simulink subsystem "Three_PhasePRController"  (R2023b)
settings: Solver=VariableStepAuto  StartTime=0.0  StopTime=10.0  RelTol=1e-3
undefined symbols (not defined in the file): prCurrentCtrl
settings Model: Creator=Veimar  LastModifiedBy=Veimar

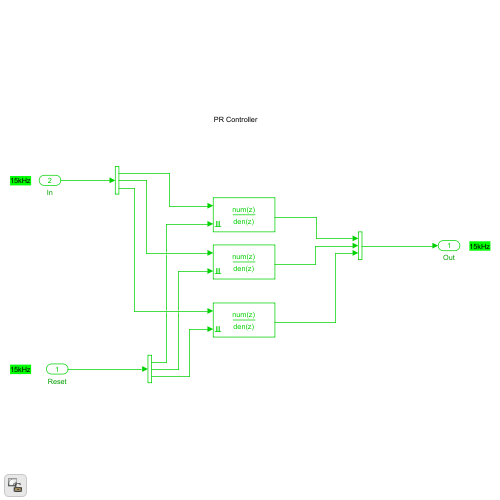
[thumbnail: Simulink's stored preview of the top-level diagram]
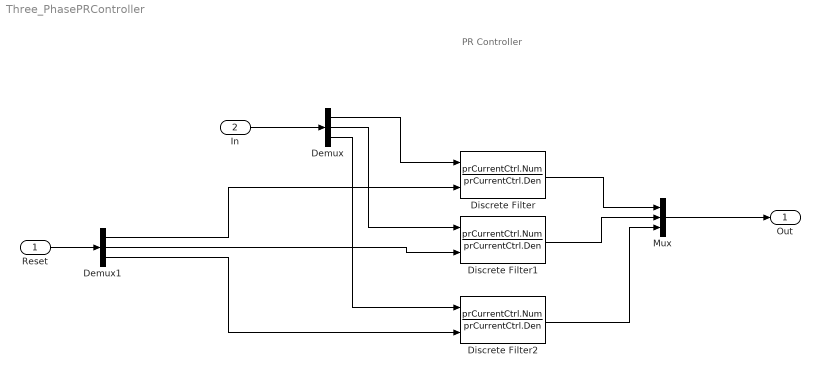
== system Three_PhasePRController ==
  note: PR Controller
  Reset : Inport
  In : Inport  Port=2
  Demux : Demux  Outputs=3
  Demux1 : Demux  Outputs=3
  Discrete Filter : DiscreteFilter  Numerator=prCurrentCtrl.Num  Denominator=prCurrentCtrl.Den  ExternalReset=Level
      settings: InputPortMap=u0,r7
  Discrete Filter1 : DiscreteFilter  Numerator=prCurrentCtrl.Num  Denominator=prCurrentCtrl.Den  ExternalReset=Level
      settings: InputPortMap=u0,r7
  Discrete Filter2 : DiscreteFilter  Numerator=prCurrentCtrl.Num  Denominator=prCurrentCtrl.Den  ExternalReset=Level
      settings: InputPortMap=u0,r7
  Mux : Mux  Inputs=3
  Out : Outport
  wires:
  In/1 -> Demux/1
  Demux/1 -> Discrete Filter/1
  Demux/2 -> Discrete Filter1/1
  Demux/3 -> Discrete Filter2/1
  Discrete Filter/1 -> Mux/1
  Discrete Filter1/1 -> Mux/2
  Discrete Filter2/1 -> Mux/3
  Mux/1 -> Out/1
  Reset/1 -> Demux1/1
  Demux1/1 -> Discrete Filter/2
  Demux1/2 -> Discrete Filter1/2
  Demux1/3 -> Discrete Filter2/2
